simulink model "Sist_stab_H"  (R2018b)
settings: Solver=VariableStepAuto  StartTime=0.0  StopTime=10.0  RelTol=1e-3
settings Model: Creator=Танечка  LastModifiedBy=Танечка

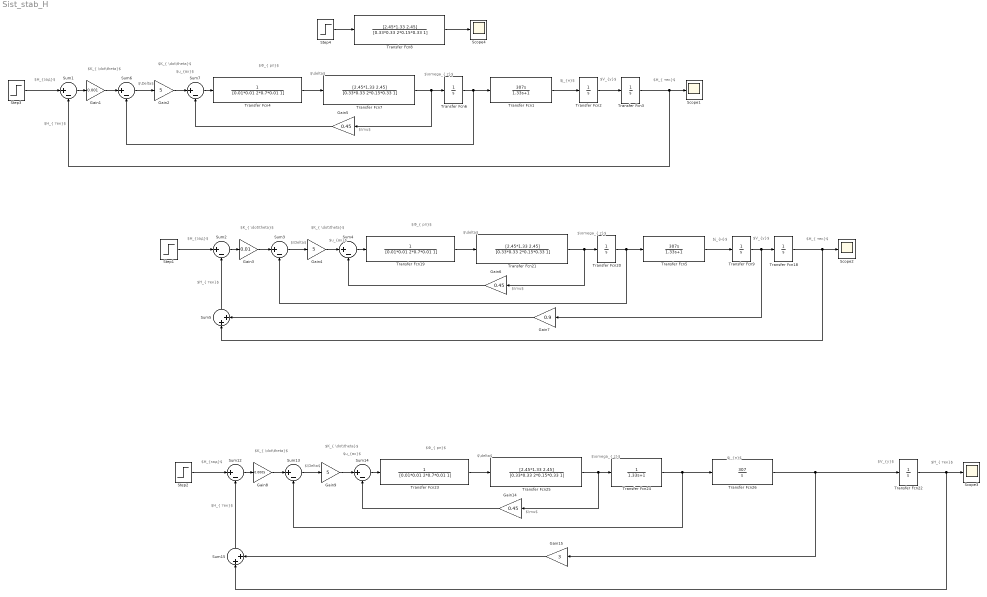
== system Sist_stab_H ==
  note: $\omega_{ z}$
  note: $\delta$
  note: $H_{ тек}$
  note: $\Delta$
  note: $u_{вх}$
  note: $K_{ \dot\theta}$
  note: $V_{y}$
  note: $H_{зад}$
  note: $\mu$
  note: $H_{ тек}$
  note: $K_{ \dot\theta}$
  note: $\Delta$
  note: $K_{ \dot\theta}$
  note: $K_{ \dot\theta}$
  note: $H_{зад}$
  note: $K_{ \dot\theta}$
  note: $Ф_{ рп}$
  note: $Ф_{ рп}$
  note: $H_{ тек}$
  note: $\omega_{ z}$
  note: $H_{ тек}$
  note: $H_{ тек}$
  note: $\mu$
  note: $V_{y}$
  note: $V_{y}$
  note: $Ф_{ рп}$
  note: $\Delta$
  note: $\omega_{ z}$
  note: $H_{ тек}$
  note: $j_{н}$
  note: $j_{н}$
  note: $u_{вх}$
  note: $\delta$
  note: $\mu$
  note: $\delta$
  note: $H_{зад}$
  note: $j_{н}$
  note: $K_{ \dot\theta}$
  note: $u_{вх}$
  Gain1 : Gain  Gain=0.001
  Gain14 : Gain  Gain=0.45
  Gain15 : Gain  Gain=3
  Gain2 : Gain  Gain=5
  Gain3 : Gain  Gain=0.01
  Gain4 : Gain  Gain=5
  Gain5 : Gain  Gain=0.45
  Gain6 : Gain  Gain=0.45
  Gain7 : Gain  Gain=0.9
  Gain8 : Gain  Gain=0.0005
  Gain9 : Gain  Gain=5
  Scope{1..4} (4 alike) : Scope
  Step1 : Step  SampleTime=0
  Step2 : Step  SampleTime=0
  Step3 : Step  SampleTime=0
  Step4 : Step  After=5  SampleTime=0
  Sum{1..4,6..7,12..14} (9 alike) : Sum  Inputs=|+-
  Sum15 : Sum  Inputs=|++
  Sum5 : Sum  Inputs=|++
  Transfer Fcn1 : TransferFcn  Numerator=[307 0]  Denominator=[1.33 1]
  Transfer Fcn{2..3,6,9,18,20,22} (7 alike) : TransferFcn  Denominator=[1 0]
  Transfer Fcn19 : TransferFcn  Numerator=[ 1]  Denominator=[0.01*0.01 2*0.7*0.01 1]
  Transfer Fcn{7..8,21,25} (4 alike) : TransferFcn  Numerator=[2.45*1.33 2.45]  Denominator=[0.33*0.33 2*0.15*0.33 1]
  Transfer Fcn23 : TransferFcn  Numerator=[ 1]  Denominator=[0.01*0.01 2*0.7*0.01 1]
  Transfer Fcn24 : TransferFcn  Denominator=[1.33 1]
  Transfer Fcn26 : TransferFcn  Numerator=[307]  Denominator=[1 0]
  Transfer Fcn4 : TransferFcn  Numerator=[ 1]  Denominator=[0.01*0.01 2*0.7*0.01 1]
  Transfer Fcn5 : TransferFcn  Numerator=[307 0]  Denominator=[1.33 1]
  wires:
  Sum12/1 -> Gain8/1
  Sum5/1 -> Sum2/2
  Sum2/1 -> Gain3/1
  Transfer Fcn18/1 -> Sum5/1, Scope2/1
  Sum4/1 -> Transfer Fcn19/1
  Transfer Fcn26/1 -> Transfer Fcn22/1, Gain15/1
  Transfer Fcn21/1 -> Gain6/1, Transfer Fcn20/1
  Sum1/1 -> Gain1/1
  Gain8/1 -> Sum13/1
  Sum14/1 -> Transfer Fcn23/1
  Gain1/1 -> Sum6/1
  Transfer Fcn22/1 -> Sum15/1, Scope3/1
  Sum13/1 -> Gain9/1
  Transfer Fcn23/1 -> Transfer Fcn25/1
  Sum3/1 -> Gain4/1
  Sum15/1 -> Sum12/2
  Transfer Fcn1/1 -> Transfer Fcn2/1
  Step2/1 -> Sum12/1
  Gain7/1 -> Sum5/2
  Gain14/1 -> Sum14/2
  Transfer Fcn8/1 -> Scope4/1
  Transfer Fcn6/1 -> Transfer Fcn1/1, Sum6/2
  Gain9/1 -> Sum14/1
  Transfer Fcn4/1 -> Transfer Fcn7/1
  Transfer Fcn25/1 -> Gain14/1, Transfer Fcn24/1
  Transfer Fcn24/1 -> Transfer Fcn26/1, Sum13/2
  Gain15/1 -> Sum15/2
  Transfer Fcn9/1 -> Gain7/1, Transfer Fcn18/1
  Transfer Fcn19/1 -> Transfer Fcn21/1
  Transfer Fcn2/1 -> Transfer Fcn3/1
  Transfer Fcn20/1 -> Transfer Fcn5/1, Sum3/2
  Step1/1 -> Sum2/1
  Transfer Fcn5/1 -> Transfer Fcn9/1
  Sum6/1 -> Gain2/1
  Transfer Fcn3/1 -> Sum1/2, Scope1/1
  Gain6/1 -> Sum4/2
  Gain2/1 -> Sum7/1
  Transfer Fcn7/1 -> Gain5/1, Transfer Fcn6/1
  Step4/1 -> Transfer Fcn8/1
  Gain5/1 -> Sum7/2
  Gain4/1 -> Sum4/1
  Step3/1 -> Sum1/1
  Sum7/1 -> Transfer Fcn4/1
  Gain3/1 -> Sum3/1
